simulink model "Arquitecture_1_Parallel_EXP"  (Simulink 8.1)
settings: Solver=ode3  StartTime=0.0  StopTime=1  FixedStep=1  RelTol=1e-3
undefined symbols (not defined in the file or in its folder): cacode, i, magnitude
libraries: dspxfrm3 x6, dspmtrx3 x4, UndergraduateResearch x3, dspstat3 x2, dspindex x1, dspsigattribs x1, simulink x1
settings Model: Creator=Willyvon  LastModifiedBy=dmiralles
settings DebuggingCC: FcnCallInpInsideContextMsg=EnableAllAsWarning
settings GRTTargetCC: CombineOutputUpdateFcns=on  GRTInterface=off

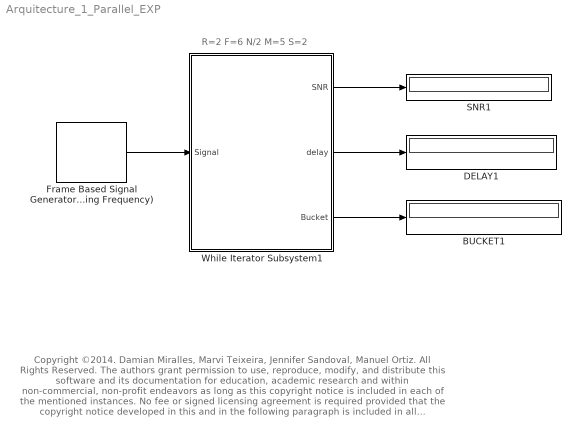
== system Arquitecture_1_Parallel_EXP ==
  note: R=2 F=6 N/2 M=5 S=2
  note: Copyright ©2014.  Damian Miralles, Marvi Teixeira, Jennifer Sandoval, Manuel Ortiz. All Rights Reserved.
      | The authors grant permission to use, reproduce, modify, and distribute this software and its documentation for
      | education,  academic research and within non-commercial, non-profit endeavors as long as this copyright notice
      |  is included in each of the mentioned instances. No fee or signed licensing agreement is required provided that
      | the copyright notice developed in this and in the following  paragraph is included in all reproductions,  alterations,
      | and distributions of the software or its  documentation. Contact the authors regarding any commercial licensing needs.
      |
      | THIS EXPERIMENTAL SOFTWARE AND RELATED DOCUMENTATION ARE PROVIDED “AS IS” AND
      |  NO, EXPLICIT OR IMPLICT, CLAIMS REGARDING THEIR ACCURACY OR SUITABILITY ARE MADE.
      | USERS ARE RESPONSIBLE FOR SOFTWARE VALIDATION REGARDING THEIR PARTICULAR
      |  APPLICATION. NO UPDATES WILL BE OFFERED. VERY LIMITED SUPPORT COULD BE PROVIDED,
      |  BUT NOT GUARANTEED, ON A CASE BY CASE BASIS, DEPENDING ON THE AVAILABLE TIME
      |  RESOURCES AT THE TIME OF THE REQUEST.
      | (dmiralles2009@gmail.com,  cc: mteixeir@ieee.org )
  BUCKET1 : Display
  DELAY1 : Display
  Frame Based Signal Generator (Any Sampling Frequency) : UndergraduateResearch/Frame Based Signal Generator (Any Sampling Frequency)  satellites=[1 3 7 19 20 22 24 28 31]  d1=378  interference=[80 80 130 5 280 40 30 100 300]  gain="[0.2 0.7  2  3  0.3  0.9 4 1 3]"  snr=-20  fs=1023000
  SNR1 : Display
  While Iterator Subsystem1 : Subsystem  TreatAsAtomicUnit=on
  wires:
  While Iterator Subsystem1/1(SNR) -> SNR1/1
  While Iterator Subsystem1/3(Bucket) -> BUCKET1/1
  While Iterator Subsystem1/2(delay) -> DELAY1/1
  Frame Based Signal Generator (Any Sampling Frequency)/1 -> While Iterator Subsystem1/1(Signal)

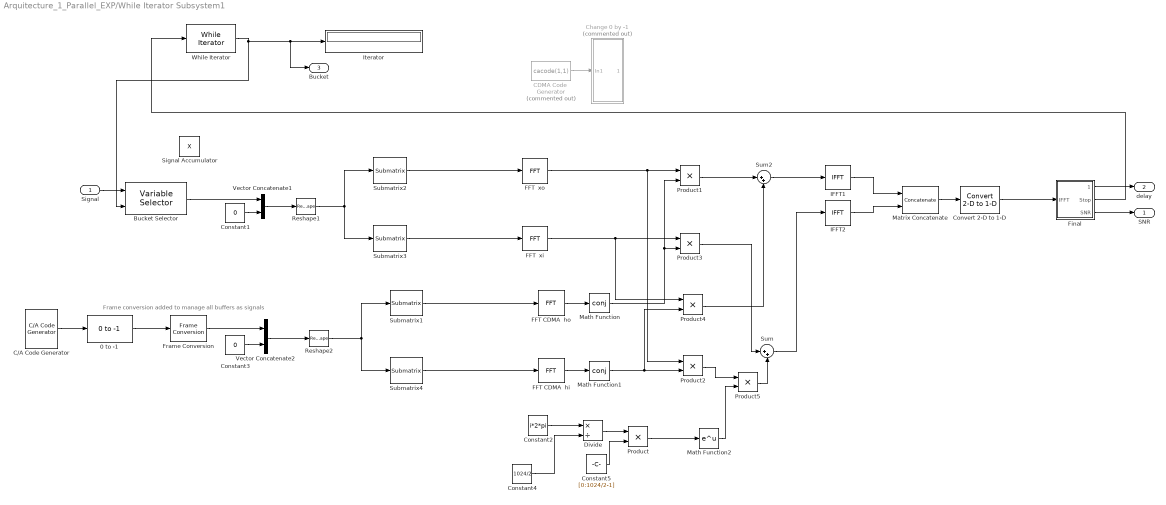
== system Arquitecture_1_Parallel_EXP/While Iterator Subsystem1 ==
  note: Frame conversion added to
      | manage all buffers as signals
  Signal : Inport
  " 0 to -1" : UndergraduateResearch/ 0 to -1
  Bucket Selector : dspindex/Variable Selector  NumInputs=1  rowsOrCols=Rows  IdxMode=Variable  Elements=[1 3]  ZerOneIdxMode=One-based  errmode=Clip Index  FillMode=on  FillValues=0
  C/A Code Generator : UndergraduateResearch/C//A Code Generator  fs=1023000  sat=1
  CDMA Code  Generator : MATLABFcn  Commented=on  MATLABFcn=cacode(1,1)  OutputDimensions=1023  Output1D=off
  Change 0 by -1 : Subsystem  Commented=on
  Constant1 : Constant  Value=0
  Constant2 : Constant  Value=i*2*pi
  Constant3 : Constant  Value=0
  Constant4 : Constant  Value=1024/2
  Constant5 : Constant  Value=[0:1024/2-1]
  Convert 2-D to 1-D : dspsigattribs/Convert 2-D to 1-D
  Divide : Product  Inputs=*/
  FFT CDMA  hi : dspxfrm3/FFT  CompMethod=Table lookup  TableOpt=NEW  TableOptActive=Speed  BitRevOrder=off  InheritFFTLength=on  FFTLength=512  RowConvenienceOn=on  FFTImplementation=FFTW  SkipNorm=off  firstCoeffDataTypeStr=Inherit: Same word length as input  firstCoeffLastDataTypeStr=Inherit: Same word length as input  outputMin=[]  outputMax=[]  roundingMode=Floor  overflowMode=off
  FFT CDMA  ho : dspxfrm3/FFT  CompMethod=Table lookup  TableOpt=NEW  TableOptActive=Speed  BitRevOrder=off  InheritFFTLength=on  FFTLength=512  RowConvenienceOn=on  FFTImplementation=FFTW  SkipNorm=off  firstCoeffDataTypeStr=Inherit: Same word length as input  firstCoeffLastDataTypeStr=Inherit: Same word length as input  outputMin=[]  outputMax=[]  roundingMode=Floor  overflowMode=off
  FFT  xi : dspxfrm3/FFT  CompMethod=Table lookup  TableOpt=NEW  TableOptActive=Speed  BitRevOrder=off  InheritFFTLength=on  FFTLength=512  RowConvenienceOn=on  FFTImplementation=FFTW  SkipNorm=off  firstCoeffDataTypeStr=Inherit: Same word length as input  firstCoeffLastDataTypeStr=Inherit: Same word length as input  outputMin=[]  outputMax=[]  roundingMode=Floor  overflowMode=off
  FFT  xo : dspxfrm3/FFT  CompMethod=Table lookup  TableOpt=NEW  TableOptActive=Speed  BitRevOrder=off  InheritFFTLength=on  FFTLength=512  RowConvenienceOn=on  FFTImplementation=FFTW  SkipNorm=off  firstCoeffDataTypeStr=Inherit: Same word length as input  firstCoeffLastDataTypeStr=Inherit: Same word length as input  outputMin=[]  outputMax=[]  roundingMode=Floor  overflowMode=off
  Final : Subsystem
      mask help:
      | The Final block receives an IFFT and returns if the SNR passed the threshhold
      | and also outputs the SNR and the delay. It uses a variable to accumulate the signal
      | adds it to IFFT and stores it. It detects the maximum value in the signal with the index and assings a 0
      | to remove the peak to be able to calculate the mean and obtain the SNR.
  Frame Conversion : FrameConversion  OutFrame=Sample-based
  IFFT1 : dspxfrm3/IFFT  CompMethod=Table lookup  TableOpt=NEW  TableOptActive=Speed  BitRevOrder=off  cs_in=off  SkipNorm=on  InheritFFTLength=on  FFTLength=512  mode=Complex  outSamplingMode=Sample based  RowConvenienceOn=on  FFTImplementation=FFTW  firstCoeffDataTypeStr=Inherit: Same word length as input  firstCoeffLastDataTypeStr=Inherit: Same word length as input  outputMin=[]  outputMax=[]  roundingMode=Floor  overflowMode=off
  IFFT2 : dspxfrm3/IFFT  CompMethod=Table lookup  TableOpt=NEW  TableOptActive=Speed  BitRevOrder=off  cs_in=off  SkipNorm=on  InheritFFTLength=on  FFTLength=512  mode=Complex  outSamplingMode=Sample based  RowConvenienceOn=on  FFTImplementation=FFTW  firstCoeffDataTypeStr=Inherit: Same word length as input  firstCoeffLastDataTypeStr=Inherit: Same word length as input  outputMin=[]  outputMax=[]  roundingMode=Floor  overflowMode=off
  Iterator : Display
  Math Function : Math  Operator=conj  SaturateOnIntegerOverflow=on
  Math Function1 : Math  Operator=conj  SaturateOnIntegerOverflow=on
  Math Function2 : Math  SaturateOnIntegerOverflow=on
  Matrix Concatenate : Concatenate  Mode=Multidimensional array
  Product{,1..5} (6 alike) : Product  RndMeth=Zero
  Reshape1 : Reshape  OutputDimensionality=Customize  OutputDimensions=[2,512]
  Reshape2 : Reshape  OutputDimensionality=Customize  OutputDimensions=[2,512]
  Signal Accumulator : DataStoreMemory  DataStoreName=X  ReadBeforeWriteMsg=warning  WriteAfterWriteMsg=warning  WriteAfterReadMsg=warning  InitialValue=zeros(1,1024)  VectorParams1D=off
  Submatrix1 : dspmtrx3/Submatrix  RowSpan=One row  RowStartMode=First  RowStartIndex=1  RowEndMode=Last  RowEndIndex=1  ColSpan=All columns  ColStartMode=First  ColStartIndex=1  ColEndMode=Last  ColEndIndex=1
  Submatrix2 : dspmtrx3/Submatrix  RowSpan=One row  RowStartMode=First  RowStartIndex=1  RowEndMode=Last  RowEndIndex=1  ColSpan=All columns  ColStartMode=First  ColStartIndex=1  ColEndMode=Last  ColEndIndex=1
  Submatrix3 : dspmtrx3/Submatrix  RowSpan=One row  RowStartMode=Last  RowStartIndex=1  RowEndMode=Last  RowEndIndex=1  ColSpan=All columns  ColStartMode=First  ColStartIndex=1  ColEndMode=Last  ColEndIndex=1
  Submatrix4 : dspmtrx3/Submatrix  RowSpan=One row  RowStartMode=Last  RowStartIndex=1  RowEndMode=Last  RowEndIndex=1  ColSpan=All columns  ColStartMode=First  ColStartIndex=1  ColEndMode=Last  ColEndIndex=1
  Sum : Sum  Inputs=|++
  Sum2 : Sum  Inputs=|++
  Vector Concatenate1 : Concatenate
  Vector Concatenate2 : Concatenate
  While Iterator : WhileIterator  MaxIters=40  WhileBlockType=do-while  ShowIterationPort=on  OutputDataType=double
  SNR : Outport
  delay : Outport  Port=2
  Bucket : Outport  Port=3  OutDataTypeStr=double
  wires:
  While Iterator/1 -> Iterator/1, Bucket/1, Bucket Selector/2
  FFT CDMA  hi/1 -> Math Function1/1
  FFT CDMA  ho/1 -> Math Function/1
  FFT  xi/1 -> Product3/1, Product4/1
  Sum2/1 -> IFFT1/1
  Constant1/1 -> Vector Concatenate1/2
  Constant3/1 -> Vector Concatenate2/2
  Bucket Selector/1 -> Vector Concatenate1/1
  FFT  xo/1 -> Product1/1, Product2/1
  Math Function/1 -> Product1/2, Product3/2
  Math Function1/1 -> Product2/2, Product4/2
  Product1/1 -> Sum2/1
  Product4/1 -> Sum2/2
  Product3/1 -> Sum/1
  Sum/1 -> IFFT2/1
  Vector Concatenate2/1 -> Reshape2/1
  Product5/1 -> Sum/2
  Product2/1 -> Product5/1
  Constant2/1 -> Divide/1
  Constant4/1 -> Divide/2
  Divide/1 -> Product/1
  Math Function2/1 -> Product5/2
  Reshape1/1 -> Submatrix3/1, Submatrix2/1
  Submatrix2/1 -> FFT  xo/1
  Submatrix3/1 -> FFT  xi/1
  Vector Concatenate1/1 -> Reshape1/1
  Reshape2/1 -> Submatrix4/1, Submatrix1/1
  Submatrix1/1 -> FFT CDMA  ho/1
  Submatrix4/1 -> FFT CDMA  hi/1
  Matrix Concatenate/1 -> Convert 2-D to 1-D/1
  IFFT1/1 -> Matrix Concatenate/1
  IFFT2/1 -> Matrix Concatenate/2
  Convert 2-D to 1-D/1 -> Final/1(IFFT)
  Constant5/1 -> Product/2
  Final/2(Stop) -> While Iterator/1
  Final/3("SNR ") -> SNR/1
  Final/1(Delay) -> delay/1
  Signal/1 -> Bucket Selector/1
  Product/1 -> Math Function2/1
  CDMA Code  Generator/1 -> Change 0 by -1/1(In1)
  C/A Code Generator/1 -> " 0 to -1"/1
  " 0 to -1"/1 -> Frame Conversion/1
  Frame Conversion/1 -> Vector Concatenate2/1

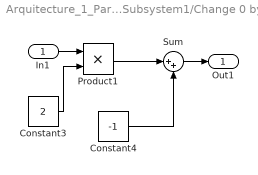
== system Arquitecture_1_Parallel_EXP/While Iterator Subsystem1/Change 0 by -1 ==
  In1 : Inport
  Constant3 : Constant  Value=2
  Constant4 : Constant  Value=-1
  Product1 : Product  RndMeth=Zero
  Sum : Sum  Inputs=|++
  Out1 : Outport
  wires:
  Product1/1 -> Sum/1
  Constant4/1 -> Sum/2
  In1/1 -> Product1/1
  Sum/1 -> Out1/1
  Constant3/1 -> Product1/2

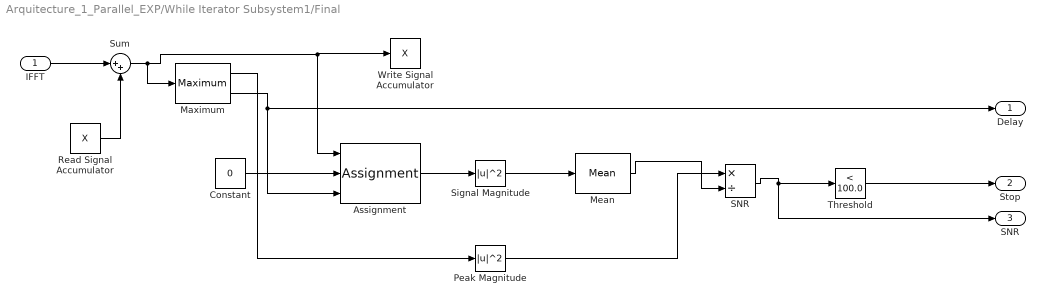
== system Arquitecture_1_Parallel_EXP/While Iterator Subsystem1/Final ==
  IFFT : Inport
  " Read Signal Accumulator" : DataStoreRead  DataStoreName=X
  Assignment : Assignment  IndexOptions=Index vector (port)  Indices=1  OutputSizes=1
  Constant : Constant  Value=0
  Maximum : dspstat3/Maximum  fcn=Value and Index  reset=None  InputProcessing=Columns as channels (frame based)  indexBase=One  operateOver=Each column  Dimension=1  colComp=on  operation=maximum  roiEnable=off  roiType=Rectangles  roiPortion=Entire ROI  roiOutput=Individual statistics for each ROI  roiFlag=off  accumDataTypeStr=Inherit: Same as product output  accumLastDataTypeStr=Inherit: Same as product output  roundingMode=Floor  overflowMode=off
  Mean : dspstat3/Mean  run=off  reset_popup=None  InputProcessing=Columns as channels (frame based)  directionMode=Each column  dimension=1  treatSBRowAsCol=on  roiEnable=off  roiType=Rectangles  roiPortion=Entire ROI  roiOutput=Individual statistics for each ROI  roiFlag=off  outputDataTypeStr=Inherit: Same as accumulator  outputLastDataTypeStr=Inherit: Same as accumulator  outputMin=[]  outputMax=[]  roundingMode=Floor  overflowMode=off
  Peak Magnitude : Math  Operator=magnitude^2  SaturateOnIntegerOverflow=on
  SNR : Product  Inputs=*/
  Signal Magnitude : Math  Operator=magnitude^2  SaturateOnIntegerOverflow=on
  Sum : Sum  Inputs=|++
  Threshold : simulink/Logic and Bit Operations/Compare To Constant  relop=<  const=100.0  OutDataTypeStr=boolean
  Write Signal Accumulator : DataStoreWrite  DataStoreName=X
  Delay : Outport
  Stop : Outport  Port=2
  "SNR " : Outport  Port=3
  wires:
  Threshold/1 -> Stop/1
  IFFT/1 -> Sum/1
  Maximum/1 -> Peak Magnitude/1
  Maximum/2 -> Delay/1, Assignment/3
  Mean/1 -> SNR/2
  SNR/1 -> "SNR "/1, Threshold/1
  Sum/1 -> Maximum/1, Assignment/1, Write Signal Accumulator/1
  " Read Signal Accumulator"/1 -> Sum/2
  Assignment/1 -> Signal Magnitude/1
  Signal Magnitude/1 -> Mean/1
  Peak Magnitude/1 -> SNR/1
  Constant/1 -> Assignment/2
